simulink model "Sim_Unknown_Constant_Gain_iqctest1"  (Simulink 7.3)
settings: Solver=ode45  StartTime=0.0  StopTime=30.0  RelTol=1e-3
settings Model: Creator=MD710  LastModifiedBy=MD710
settings DebuggingCC: SaveWithParameterizedLinksMsg=none  SolverPrmCheckMsg=none  MultiTaskDSMMsg=warning  MultiTaskCondExecSysMsg=none  FcnCallInpInsideContextMsg=Enable All  StrictBusMsg=None
settings HardwareCC: TargetHWDeviceType=32-bit Generic
settings RTWCC: IncludeERTFirstTime=on
settings GRTTargetCC: TargetFcnLib=ansi_tfl_tmw.mat

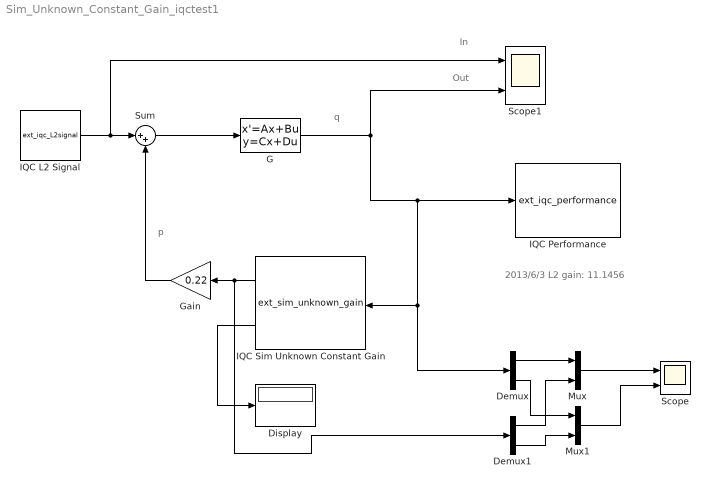
== system Sim_Unknown_Constant_Gain_iqctest1 ==
  note: q
  note: p
  note: 2013/6/3 L2 gain: 11.1456
  note: In
  note: Out
  Demux : Demux  Outputs=2
  Demux1 : Demux  Outputs=2
  Display : Display
  G : StateSpace  A=[-(-0.3+0.8*2.5*0.86) -0.8*2.5;1 0]  B=[-2 -2*0.8;0 0]  C=[-0.3+0.8*2.5*0.86 0.8*2.5;2.5*0.86 2.5]  D=[1 2*0.8;0 1]
  Gain : Gain  Gain=0.22
  IQC L2 Signal : M-S-Function  FunctionName=ext_iqc_L2signal  Parameters=sig_size,sam_time,sig_type,tru_time,sig_amp,sig_fre,user_cus  mask(IQC L2 signal(ver:0.1)){sig_size=2, sam_time=0, sig_type=Step, tru_time=10, sig_amp=1, sig_fre=1, user_cus='2*exp(3*t)'}
      mask prompts: sig_size "Signal Dimension:(Default: 1)"; sam_time "Sample Time:(Default: 0)"; sig_type "Signal Type:"; tru_time "Truncation Time:"; sig_amp "Maximum Amplitude:"; sig_fre "Frequency:"; user_cus "Custom:"
      mask help:
      | Important:
      | In IQC procedure step (as commond iqc_gain_tbx, the task is get
      | L2 gain value), regardless of the user to choose which option (ex sine...),
      | here regarded as generalized L2 signal.
      mask StyleString: edit,edit,popup(Step|Square wave|Sine wave|Custom|Random|External),edit,edit,edit,edit
      mask CallbackString: ||iqc_block_cho(gcb,'L2signal_type')||||
      mask TabNameString: Main,Main,Simulation,Simulation,Simulation,Simulation,Simulation
      mask Display: plot(0:0.1:10,[sin(0:0.1:6.2) zeros(1,38)])
  IQC Performance : M-S-Function  FunctionName=ext_iqc_performance  Parameters=imp_met,save_lin_com,isiqcbode,fre_ran,uselmitool,lmi_par  mask(IQC Performance(ver:0.1)){imp_met=Calculation and Simulation, save_lin_com=off, isiqcbode=off, fre_ran='', uselmitool=lmilab, lmi_par=''}
      mask prompts: imp_met "Implementation Methods"; save_lin_com "Save the Linear File and Command File"; isiqcbode "Display IQC Bode Figure"; fre_ran "Frequency Range:(Default: empty)"; uselmitool "LMI Tool:"; lmi_par "Parameter:(if empty use define)"
      mask help:
      | Important:
      | In IQC toolbox calculate step (as commond iqc_gain_tbx, the task is get
      | L2 gain value), regardless of the user to connect any signal input(Even if
      | not a signal), here regarded as generalized L2 signal.
      |
      | Example 1: setlmioptions('',[0 200 0 0 777])
      | the block parameter is
      | LMI Tool: lmilab
      | Parameter:
      |        [0 200 0 0 777]
      |
      | Example 2: setlmioptions('yalmip','solver','sdpt3','verbose',1)
      | the block parameter is
      | LMI Tool: yalmip
      | Parameter:
      |        {'solver',sdpt3','verbose',1}
      mask Help:
      | <a href="matlab:doc abst_init_iqc;">abst_init_iqc</a>
      | <a href="matlab:doc setlmioptions;">setlmioptions</a>
      | <a href="matlab:doc iqc_gain_tbx;">iqc_gain_tbx</a>
      mask StyleString: popup(Calculation and Simulation|Only Calculation|Only Simulation),checkbox,checkbox,edit,popup(lmilab|yalmip),edit
      mask CallbackString: iqc_block_cho(gcb,'performance_imp')||iqc_block_cho(gcb,'performance_bodefre')|||
      mask TabNameString: Main,Main,Main,Main,LMI,LMI
      mask Display: fprintf('In -> Out \n performance \n L2 gain:\n%4.4f',11.1456);
  IQC Sim Unknown Constant Gain : M-S-Function  FunctionName=ext_sim_unknown_gain  Parameters=sou_con,num_ran,cus,iqc1,iqc1_pole,iqc1_out,iqc2,iqc2_out,iqc3,iqc3_out,iqc4,lis_rel,rand_cons  mask(IQC Sim Unknown Constant Gain(ver:0.1)){sou_con=Random, num_ran=2, cus=[0.3], iqc1=on, iqc1_pole=[1], iqc1_out='', iqc2=off, iqc2_out='', iqc3=off, iqc3_out='', iqc4=off, lis_rel='', rand_cons=0}
      mask prompts: sou_con "Source of The Constant Gain:(Default: Random)"; num_ran "The Number of Random:(1 or input_dim)"; cus "Custom:"; iqc1 "iqc_ltigain(Input,Pole)"; iqc1_pole "Pole:(Default: [1])"; iqc1_out "Output Variable:(Default: empty)"; iqc2 "iqc_ltvnorm(Input,length(Input),1)"; iqc2_out "Output Variable:(Default: empty)"; iqc3 "iqc_tvscalar(Input,1)"; iqc3_out "Output Variable:(Default: empty)"; iqc4 "Custom IQC"; lis_rel "List of IQC Relationships:"; rand_cons "Mask Parameter 13:"
      mask init:
      | switch sou_con
      |     case 1
      |         rand_cons=rand(1,num_ran);
      |     case 2
      |         if any(abs(cus)>1)
      |             error('the maximum random constant is 1')
      |         else
      |             rand_cons=reshape(cus,1,length(cus));
      |         end
      | end
      mask Help:
      | <a href="matlab:doc iqc_ltigain;">iqc_ltigain</a>
      | <a href="matlab:doc iqc_ltvnorm;">iqc_ltvnorm</a>
      | <a href="matlab:doc iqc_tvscalar;">iqc_tvscalar</a>
      mask StyleString: popup(Random|Custom),edit,edit,checkbox,edit,edit,checkbox,edit,checkbox,edit,checkbox,edit,edit
      mask CallbackString: iqc_block_cho(gcb,'sim_constantgain_sou')|||iqc_block_cho(gcb,'sim_constantgain_iqc1')|||iqc_block_cho(gcb,'sim_constantgain_iqc2')||iqc_block_cho(gcb,'sim_constantgain_iqc3')||iqc_block_cho(gcb,'sim_constantgain_iqc4')||
      mask TabNameString: Simulink Parameters,Simulink Parameters,Simulink Parameters,Procedure Parameters,Procedure Parameters,Procedure Parameters,Procedure Parameters,Procedure Parameters,Procedure Parameters,Procedure Parameters,Procedure Parameters,Procedure Parameters,Simulink Parameters
      mask Display: disp('\fontsize{14}|d| < 1', 'texmode','on');port_label('input',1,'in');port_label('output',1,'out');port_label('output',2,'|d|');
  Mux : Mux  Inputs=2
  Mux1 : Mux  Inputs=2
  Scope : Scope  NumInputPorts=2
      settings: YMin=-5~-5  YMax=5~5
  Scope1 : Scope  NumInputPorts=2
      settings: YMin=-5~-5  YMax=5~5
  Sum : Sum  Inputs=|++
  wires:
  IQC L2 Signal/1 -> Scope1/1, Sum/1
  Sum/1 -> G/1
  G/1 -> IQC Performance/1, Demux/1, IQC Sim Unknown Constant Gain/1, Scope1/2
  Gain/1 -> Sum/2
  IQC Sim Unknown Constant Gain/1 -> Demux1/1, Gain/1
  IQC Sim Unknown Constant Gain/2 -> Display/1
  Demux/1 -> Mux/1
  Demux1/1 -> Mux/2
  Mux/1 -> Scope/1
  Demux/2 -> Mux1/1
  Demux1/2 -> Mux1/2
  Mux1/1 -> Scope/2
